simulink model "Mod1_2d_VyP"  (R2019a)
settings: Solver=VariableStepAuto  StartTime=0.0  StopTime=370  MaxStep=0.01  RelTol=1e-3
values from neighbouring files (symbols this model uses):
  a_s = 0.32    [Mod1_2d_VyP_pars.m]
settings Model: Creator=Luis F Guevara G  LastModifiedBy=Luis F Guevara G

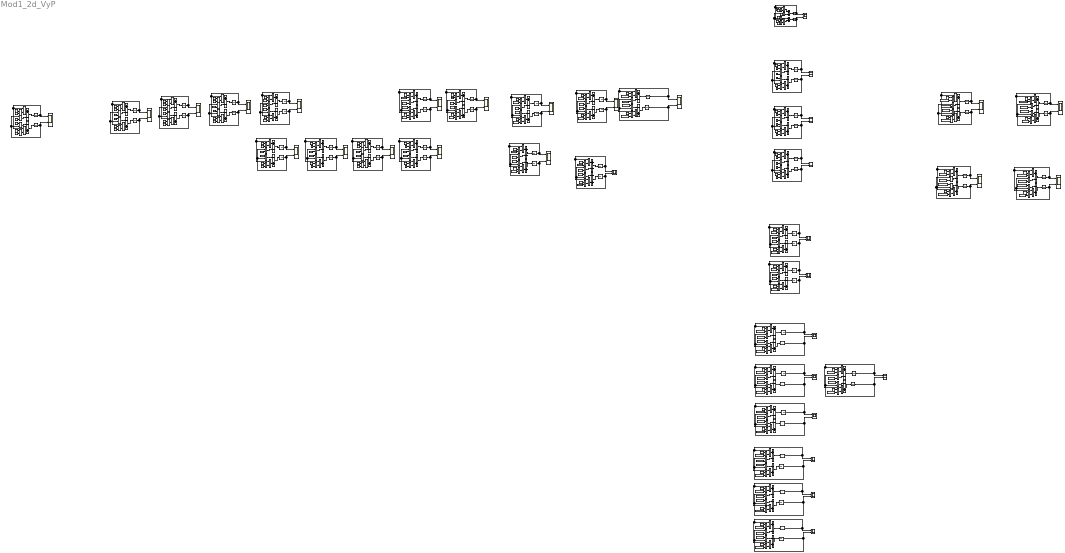
== system Mod1_2d_VyP ==
  note: ESTOS SON DE LOS USADOS
      | PARA EL DOCUMENTO DE LA TESIS
  note: CONSIDEREMOS DATOS DE FERNANDA PARTO #3
      | Peso inicial 515 (Integrador arriba)
      | Desperdicio inicial 44.75 (Integrador abajo)
  note: Cómo controlo la llegada al maximo para
      | luego cambiar el control al llegar al minimo
      | Toca usar automata? omg
  note: OJO SUPER OJO AQUI
  note: Con estos valores, logramos un crecimiento hasta punto maximo
      | y luego decrecimiento hasta que se hace 0
  note: K1=1
      | K2=1
      | K3=1
      | K4= 1
      | a_s = 0.32
  note: P
  note: W
  note: K1=1
      | K2=0.5
      | K3=1
      | K4=0.5
      | a_s = 0.32
  note: P
  note: W
  note: K1=1
      | K2=0.5
      | K3=1
      | K4=0.5
      | a_s = 0.32
  note: P
  note: W
  note: K1=0.5
      | K2=0.25
      | K3=0.5
      | K4=0.25
      | a_s = 0.32
  note: P
  note: W
  note: P
  note: W
  note: K1=1
      | K2=0.3
      | K3=1
      | K4=0.3
      | a_s = 0.32
  note: P
  note: W
  note: K1=1
      | K2=0.51
      | K3=1
      | K4=0.5
      | a_s = 0.32
  note: P
  note: W
  note: Si k4 es mayor a k2 (doble, se indetermina a infinito)
  note: K1=1
      | K2=0.51
      | K3=1
      | K4=0.511
      | a_s = 0.32
  note: OJO SUPER OJO AQUI
  note: Con estos valores, logramos un crecimiento hasta punto maximo
      | y luego decrecimiento hasta que se hace 0
  note: P
  note: W
  note: K1=1
      | K2=0.51
      | K3=1
      | K4=0.509
      | a_s = 0.32
  note: Cómo controlo la llegada al maximo para
      | luego cambiar el control al llegar al minimo
      | Toca usar automata? omg
  note: Con estos valores, logramos un crecimiento hasta punto maximo
      | y luego decrecimiento hasta que se hace 0
  note: W
  note: Cómo controlo la llegada al maximo para
      | luego cambiar el control al llegar al minimo
      | Toca usar automata? omg
  note: OJO SUPER OJO AQUI
  note: P
  note: K1=1
      | K2=0.3
      | K3=1
      | K4=0.29
      | a_s = 0.32
  note: Cómo controlo la llegada al maximo para
      | luego cambiar el control al llegar al minimo
      | Toca usar automata? omg
  note: OJO SUPER OJO AQUI
  note: P
  note: Con estos valores, logramos un crecimiento hasta punto maximo
      | y luego decrecimiento hasta que se hace 0
  note: W
  note: K1=1
      | K2=0.4
      | K3=1
      | K4=0.39
      | a_s = 0.32
  note: W
  note: K1=1
      | K2=0.45
      | K3=1
      | K4=0.44
      | a_s = 0.32
  note: Con estos valores, logramos un crecimiento hasta punto maximo
      | y luego decrecimiento hasta que se hace 0
  note: P
  note: OJO SUPER OJO AQUI
  note: Cómo controlo la llegada al maximo para
      | luego cambiar el control al llegar al minimo
      | Toca usar automata? omg
  note: W
  note: K1=1
      | K2=0.45
      | K3=1
      | K4=0.44
      | a_s = 0.32
  note: Con estos valores, logramos un crecimiento hasta punto maximo
      | y luego decrecimiento hasta que se hace 0 POR ALLA EN T=2K
  note: P
  note: OJO SUPER OJO AQUI
  note: Cómo controlo la llegada al maximo para
      | luego cambiar el control al llegar al minimo
      | Toca usar automata? omg
  note: W
  note: K1=0.3
      | K2=0.7
      | K3=0.2975
      | K4=0.5
      | a_s = 0.32
  note: Con estos valores, logramos un crecimiento hasta punto maximo
      | y luego decrecimiento hasta que se hace 0 POR ALLA EN T=2K
  note: P
  note: OJO SUPER OJO AQUI
  note: Cómo controlo la llegada al maximo para
      | luego cambiar el control al llegar al minimo
      | Toca usar automata? omg
  note: W
  note: K1=0.3
      | K2=0.7
      | K3=0.2975
      | K4=0.5
      | a_s = 0.32
  note: Con estos valores, logramos un crecimiento hasta punto maximo
      | y luego decrecimiento hasta que se hace 0 POR ALLA EN T=2K
  note: P
  note: OJO SUPER OJO AQUI
  note: Cómo controlo la llegada al maximo para
      | luego cambiar el control al llegar al minimo
      | Toca usar automata? omg
  note: CONSIDEREMOS DATOS DE FERNANDA PARTO #3
      | Peso inicial 515 (Integrador arriba)
      | Desperdicio inicial 44.75 (Integrador abajo)
  note: Con estos valores, logramos un crecimiento hasta punto maximo
      | y luego decrecimiento hasta que se hace 0 POR ALLA EN T=2K
  note: Cómo controlo la llegada al maximo para
      | luego cambiar el control al llegar al minimo
      | Toca usar automata? omg
  note: P
  note: W
  note: OJO SUPER OJO AQUI
  note: K1=0.3
      | K2=0.7
      | K3=0.2975
      | K4=0.5
      | a_s = 0.32
  note: W
  note: K1=0.3
      | K2=0.7
      | K3=0.2975
      | K4=0.5
      | a_s = 0.32
  note: Con estos valores, logramos un crecimiento hasta punto maximo
      | y luego decrecimiento hasta que se hace 0 POR ALLA EN T=2K
  note: P
  note: OJO SUPER OJO AQUI
  note: Cómo controlo la llegada al maximo para
      | luego cambiar el control al llegar al minimo
      | Toca usar automata? omg
  note: W
  note: K1=0.3
      | K2=0.7
      | K3=0.2975
      | K4=0.5
      | a_s = 0.32
  note: Con estos valores, logramos un crecimiento hasta punto maximo
      | y luego decrecimiento hasta que se hace 0 POR ALLA EN T=2K
  note: P
  note: OJO SUPER OJO AQUI
  note: Cómo controlo la llegada al maximo para
      | luego cambiar el control al llegar al minimo
      | Toca usar automata? omg
  note: W
  note: P
  note: Parto#3 - Python
      | Fernanda
  note: W
  note: K1=0.2798
      | K2=1
      | K3=0.03218
      | K4=0.1148
      | a_s = 0.32
  note: Con estos valores, logramos un crecimiento hasta punto maximo
      | y luego decrecimiento hasta que se hace 0 POR ALLA EN T=2K
  note: P
  note: OJO SUPER OJO AQUI
  note: Cómo controlo la llegada al maximo para
      | luego cambiar el control al llegar al minimo
      | Toca usar automata? omg
  note: Parto#3 - Python
      | Guapa
  note: W
  note: K1=0.2798
      | K2=1
      | K3=0.03218
      | K4=0.1148
      | a_s = 0.32
  note: Con estos valores, logramos un crecimiento hasta punto maximo
      | y luego decrecimiento hasta que se hace 0 POR ALLA EN T=2K
  note: P
  note: OJO SUPER OJO AQUI
  note: Cómo controlo la llegada al maximo para
      | luego cambiar el control al llegar al minimo
      | Toca usar automata? omg
  note: Parto#3 - Python
      | Juana
  note: W
  note: K1=0.2798
      | K2=1
      | K3=0.03218
      | K4=0.1148
      | a_s = 0.32
  note: Con estos valores, logramos un crecimiento hasta punto maximo
      | y luego decrecimiento hasta que se hace 0 POR ALLA EN T=2K
  note: P
  note: OJO SUPER OJO AQUI
  note: Cómo controlo la llegada al maximo para
      | luego cambiar el control al llegar al minimo
      | Toca usar automata? omg
  note: Parto#3 - Python
      | Leticia
  note: W
  note: K1=0.2798
      | K2=1
      | K3=0.03218
      | K4=0.1148
      | a_s = 0.32
  note: Con estos valores, logramos un crecimiento hasta punto maximo
      | y luego decrecimiento hasta que se hace 0 POR ALLA EN T=2K
  note: P
  note: OJO SUPER OJO AQUI
  note: Cómo controlo la llegada al maximo para
      | luego cambiar el control al llegar al minimo
      | Toca usar automata? omg
  note: P
  note: W
  note: K1=1
      | K2=0.5
      | K3=1
      | K4=0.5
      | a_s = 0.32
  note: P
  note: W
  note: CONSIDEREMOS DATOS DE FERNANDA PARTO #3
      | Peso inicial 515 (Integrador arriba)
      | Desperdicio inicial 44.75 (Integrador abajo)
  note: W
  note: K1=0.3
      | K2=0.7
      | K3=0.2975
      | K4=0.5
      | a_s = 0.32
  note: Con estos valores, logramos un crecimiento hasta punto maximo
      | y luego decrecimiento hasta que se hace 0 POR ALLA EN T=2K
  note: P
  note: OJO SUPER OJO AQUI
  note: Cómo controlo la llegada al maximo para
      | luego cambiar el control al llegar al minimo
      | Toca usar automata? omg
  note: P
  note: W
  note: P
  note: W
  note: P
  note: W
  note: P
  note: W
  note: P
  note: W
  note: P
  note: W
  note: W
  note: P
  note: ESTOS SON DE LOS USADOS
      | PARA EL DOCUMENTO DE LA TESIS
  note: ESTOS SON DE LOS USADOS
      | PARA EL DOCUMENTO DE LA TESIS
  note: Corroboración del ajuste
      | de modelos Python
  note: P
  note: W
  Add{,2,4,6,8,10,12,14,16,18,20,22,24,26,28,30,32,34,36,38,40,42,44,46,48,50,52,54,56,58,60,62,64} (33 alike) : Sum  Inputs=+-
  Add{1,3,5,7,9,11,13,15,17,19,21,23,25,27,29,31,33,35,37,39,41,43,45,47,49,51,53,55,57,59,61,63,65} (33 alike) : Sum  Inputs=-+
  Constant{,1..65} (66 alike) : Constant  Value=a_s
  Integrator{,2,4,6,8,10,12,14,16,18,20,22,24,30,32,34,44,46,48,50,52,54,56,58,60,62,64} (27 alike) : Integrator  InitialCondition=400
  Integrator{1,3,5,7,9,11,13,15,17,19,21,23,25,31,33,35,45,47,49,51,53,55,57,59,61,63,65} (27 alike) : Integrator  InitialCondition=40
  Integrator26 : Integrator  InitialCondition=515
  Integrator27 : Integrator  InitialCondition=44.75
  Integrator28 : Integrator  InitialCondition=515
  Integrator29 : Integrator  InitialCondition=44.75
  Integrator36 : Integrator  InitialCondition=515
  Integrator37 : Integrator  InitialCondition=44.75
  Integrator38 : Integrator  InitialCondition=500
  Integrator39 : Integrator  InitialCondition=44
  Integrator40 : Integrator  InitialCondition=600
  Integrator41 : Integrator  InitialCondition=43.4
  Integrator42 : Integrator  InitialCondition=396
  Integrator43 : Integrator  InitialCondition=36.2
  K1 {1..2,5..12,23} (11 alike) : Constant
  K1 13 : Constant  Value=0.3
  K1 14 : Constant  Value=0.7
  K1 15 : Constant  Value=0.65
  K1 16 : Constant  Value=0.345
  K1 17 : Constant  Value=0.4475
  K1 18 : Constant  Value=0.1563
  K1 19 : Constant  Value=0.27982548
  K1 20 : Constant  Value=0.26049969
  K1 21 : Constant  Value=0.22004866
  K1 22 : Constant  Value=0.30990678
  K1 24 : Constant  Value=0.5
  K1 25 : Constant  Value=0.6
  K1 26 : Constant  Value=0.69
  K1 27 : Constant  Value=0.65
  K1 28 : Constant  Value=0.8
  K1 29 : Constant  Value=0.2
  K1 3 : Constant  Value=0.5
  K1 30 : Constant  Value=0.69
  K1 31 : Constant  Value=0.051755
  K1 32 : Constant  Value=0.95
  K1 4 : Constant  Value=0.5
  P#3 Fer : Scope  NumInputPorts=2
  P#3 Gpa : Scope  NumInputPorts=2
  P#3 Juan : Scope  NumInputPorts=2
  P#3 Leti : Scope  NumInputPorts=2
  Product{,1..197} (198 alike) : Product
  Scope{,3..16,18,20} (17 alike) : Scope  NumInputPorts=2
  igualki : Scope  NumInputPorts=2
  k1 : Constant
  k1MAPk3_k2MAPk4 : Scope  NumInputPorts=2
  k1MAPk3_k2MAPk4_k1Mk2 : Scope  NumInputPorts=2
  k1Mk2_k3Mk4 : Scope  NumInputPorts=2
  k1Mk3_k2Mk4 : Scope  NumInputPorts=2
  k1menk2_k3menk3 : Scope  NumInputPorts=2
  k1menk2_k3menk4 : Scope  NumInputPorts=2
  k1menk3_k2menk1 : Scope  NumInputPorts=2
  k1menk3_k2menk2 : Scope  NumInputPorts=2
  k1menk3_k2menk4 : Scope  NumInputPorts=2
  k2 {,1,3,19,22..23} (6 alike) : Constant
  k2 10 : Constant  Value=0.4
  k2 11 : Constant  Value=0.45
  k2 12 : Constant  Value=0.45
  k2 13 : Constant  Value=0.7
  k2 14 : Constant  Value=0.7
  k2 15 : Constant  Value=0.8
  k2 16 : Constant  Value=0.7
  k2 17 : Constant  Value=0.9
  k2 18 : Constant  Value=0.61
  k2 2 : Constant  Value=0.5
  k2 20 : Constant  Value=0.99999983
  k2 21 : Constant  Value=0.99999824
  k2 24 : Constant  Value=0.5
  k2 25 : Constant  Value=0.69
  k2 26 : Constant  Value=0.6
  k2 27 : Constant  Value=0.8
  k2 28 : Constant  Value=0.9
  k2 29 : Constant  Value=0.69
  k2 30 : Constant  Value=0.69
  k2 31 : Constant  Value=0.051
  k2 32 : Constant  Value=0.8
  k2 4 : Constant  Value=0.25
  k2 5 : Constant  Value=0.3
  k2 6 : Constant  Value=0.51
  k2 7 : Constant  Value=0.51
  k2 8 : Constant  Value=0.51
  k2 9 : Constant  Value=0.3
  k2Mk1_k3MAPk4 : Scope  NumInputPorts=2
  k3 : Constant
  k3 {1..2,5..11,23} (10 alike) : Constant
  k3 12 : Constant  Value=0.9795
  k3 13 : Constant  Value=0.2975
  k3 14 : Constant  Value=0.5
  k3 {15,27..29} (4 alike) : Constant  Value=0.6
  k3 16 : Constant  Value=0.2755
  k3 17 : Constant  Value=0.3755
  k3 18 : Constant  Value=0.051755
  k3 19 : Constant  Value=0.03218680
  k3 20 : Constant  Value=0.02688459
  k3 21 : Constant  Value=0.0169588
  k3 22 : Constant  Value=0.04221679
  k3 24 : Constant  Value=0.7
  k3 25 : Constant  Value=0.65
  k3 26 : Constant  Value=0.8
  k3 3 : Constant  Value=0.5
  k3 30 : Constant  Value=0.7
  k3 31 : Constant  Value=0.61
  k3 32 : Constant  Value=0.9
  k3 4 : Constant  Value=0.5
  k3Mk4_k1MAPk2 : Scope  NumInputPorts=2
  k4 : Constant
  k4 1 : Constant
  k4 10 : Constant  Value=0.39
  k4 11 : Constant  Value=0.44
  k4 12 : Constant  Value=0.44
  k4 {2,6,13..14,16} (5 alike) : Constant  Value=0.5
  k4 {15,27..28,32} (4 alike) : Constant  Value=0.69
  k4 17 : Constant  Value=0.7
  k4 18 : Constant  Value=0.051
  k4 19 : Constant  Value=0.11480125
  k4 20 : Constant  Value=0.10349996
  k4 21 : Constant  Value=0.07715987
  k4 22 : Constant  Value=0.13587340
  k4 23 : Constant
  k4 24 : Constant  Value=0.7
  k4 25 : Constant  Value=0.8
  k4 26 : Constant  Value=0.65
  k4 29 : Constant  Value=0.8
  k4 3 : Constant
  k4 30 : Constant  Value=0.8
  k4 31 : Constant  Value=0.051
  k4 4 : Constant  Value=0.25
  k4 5 : Constant  Value=0.3
  k4 7 : Constant  Value=0.50
  k4 8 : Constant  Value=0.511
  k4 9 : Constant  Value=0.29
  wires:
  Add/1 -> Integrator/1
  Integrator/1 -> Scope/1, Product1/1, Product6/1  "Peso"
  Integrator1/1 -> Product2/1, Product7/2, Scope/2  "Producido"
  Constant/1 -> Product/1
  K1 1/1 -> Product/2
  Product/1 -> Product1/2
  Product1/1 -> Add/1
  k2 1/1 -> Product2/2
  Product2/1 -> Add/2
  k3 1/1 -> Product5/2
  Constant7/1 -> Product5/1
  Product6/1 -> Add1/2
  Product5/1 -> Product6/2
  k4 1/1 -> Product7/1
  Product7/1 -> Add1/1
  Add1/1 -> Integrator1/1
  Add3/1 -> Integrator3/1
  Product11/1 -> Add3/1
  k4 2/1 -> Product11/1
  Product9/1 -> Product10/2
  Product10/1 -> Add3/2
  Constant2/1 -> Product9/1
  k3 2/1 -> Product9/2
  Product8/1 -> Add2/2
  k2 2/1 -> Product8/2
  Product4/1 -> Add2/1
  Product3/1 -> Product4/2
  K1 2/1 -> Product3/2
  Constant1/1 -> Product3/1
  Integrator3/1 -> k1Mk2_k3Mk4/2, Product11/2, Product8/1  "Producido"
  Integrator2/1 -> k1Mk2_k3Mk4/1, Product10/1, Product4/1  "Peso"
  Add2/1 -> Integrator2/1
  Integrator5/1 -> k1menk2_k3menk4/2, Product13/2, Product16/1  "Desp"
  Product15/1 -> Add4/1
  k2 3/1 -> Product16/2
  Add4/1 -> Integrator4/1
  k3 3/1 -> Product17/2
  Product16/1 -> Add4/2
  Constant3/1 -> Product14/1
  K1 3/1 -> Product14/2
  Product17/1 -> Product12/2
  Constant4/1 -> Product17/1
  Product14/1 -> Product15/2
  Integrator4/1 -> Product12/1, Product15/1, k1menk2_k3menk4/1  "Peso"
  Product12/1 -> Add5/2
  k4 3/1 -> Product13/1
  Product13/1 -> Add5/1
  Add5/1 -> Integrator5/1
  Integrator7/1 -> Scope3/2, Product19/2, Product22/1  "Desp"
  Product21/1 -> Add6/1
  k2 4/1 -> Product22/2
  Add6/1 -> Integrator6/1
  k3 4/1 -> Product23/2
  Product22/1 -> Add6/2
  Constant5/1 -> Product20/1
  K1 4/1 -> Product20/2
  Product23/1 -> Product18/2
  Constant6/1 -> Product23/1
  Product20/1 -> Product21/2
  Integrator6/1 -> Product18/1, Product21/1, Scope3/1  "Peso"
  Product18/1 -> Add7/2
  k4 4/1 -> Product19/1
  Product19/1 -> Add7/1
  Add7/1 -> Integrator7/1
  k4 5/1 -> Product25/1
  Product24/1 -> Add9/2
  Product25/1 -> Add9/1
  Add9/1 -> Integrator9/1
  Product26/1 -> Product27/2
  Integrator8/1 -> Product24/1, Product27/1, Scope4/1  "Peso"
  K1 5/1 -> Product26/2
  Constant9/1 -> Product29/1
  k3 5/1 -> Product29/2
  Constant8/1 -> Product26/1
  Add8/1 -> Integrator8/1
  Product28/1 -> Add8/2
  Product29/1 -> Product24/2
  k2 5/1 -> Product28/2
  Product27/1 -> Add8/1
  Integrator9/1 -> Scope4/2, Product25/2, Product28/1  "Desp"
  Integrator11/1 -> Scope5/2, Product31/2, Product34/1  "Desp"
  Constant11/1 -> Product35/1
  Add10/1 -> Integrator10/1
  k2 6/1 -> Product34/2
  k3 6/1 -> Product35/2
  Product35/1 -> Product30/2
  Product33/1 -> Add10/1
  Product34/1 -> Add10/2
  K1 6/1 -> Product32/2
  Constant10/1 -> Product32/1
  Product32/1 -> Product33/2
  Add11/1 -> Integrator11/1
  Integrator10/1 -> Product30/1, Product33/1, Scope5/1  "Peso"
  Product31/1 -> Add11/1
  k4 6/1 -> Product31/1
  Product30/1 -> Add11/2
  Product42/1 -> Add15/2
  Add14/1 -> Integrator14/1
  k2 8/1 -> Product46/2
  Product43/1 -> Add15/1
  k3 8/1 -> Product47/2
  Product45/1 -> Add14/1
  Product46/1 -> Add14/2
  K1 8/1 -> Product44/2
  Product44/1 -> Product45/2
  Constant14/1 -> Product44/1
  Add15/1 -> Integrator15/1
  Integrator15/1 -> Scope7/2, Product43/2, Product46/1  "Desp"
  Product47/1 -> Product42/2
  k4 8/1 -> Product43/1
  Integrator14/1 -> Product42/1, Product45/1, Scope7/1  "Peso"
  Constant15/1 -> Product47/1
  Add13/1 -> Integrator13/1
  Constant12/1 -> Product38/1
  Product38/1 -> Product39/2
  K1 7/1 -> Product38/2
  Product40/1 -> Add12/2
  Product39/1 -> Add12/1
  k3 7/1 -> Product41/2
  k2 7/1 -> Product40/2
  Add12/1 -> Integrator12/1
  Product41/1 -> Product36/2
  Integrator13/1 -> Scope6/2, Product37/2, Product40/1  "Desp"
  Constant13/1 -> Product41/1
  Integrator12/1 -> Product39/1, Product36/1, Scope6/1  "Peso"
  k4 7/1 -> Product37/1
  Product36/1 -> Add13/2
  Product37/1 -> Add13/1
  Integrator16/1 -> Product51/1, Product48/1, Scope8/1  "Peso"
  Constant17/1 -> Product53/1
  Product48/1 -> Add17/2
  k4 9/1 -> Product49/1
  Integrator17/1 -> Scope8/2, Product49/2, Product52/1  "Desp"
  Product53/1 -> Product48/2
  Add16/1 -> Integrator16/1
  Product49/1 -> Add17/1
  k2 9/1 -> Product52/2
  Product52/1 -> Add16/2
  k3 9/1 -> Product53/2
  K1 9/1 -> Product50/2
  Add17/1 -> Integrator17/1
  Product51/1 -> Add16/1
  Constant16/1 -> Product50/1
  Product50/1 -> Product51/2
  Add19/1 -> Integrator19/1
  Constant18/1 -> Product56/1
  Product57/1 -> Add18/1
  K1 10/1 -> Product56/2
  k2 10/1 -> Product58/2
  k3 10/1 -> Product59/2
  Product55/1 -> Add19/1
  Product58/1 -> Add18/2
  Integrator19/1 -> Scope9/2, Product55/2, Product58/1  "Desp"
  Add18/1 -> Integrator18/1
  Product59/1 -> Product54/2
  Product54/1 -> Add19/2
  k4 10/1 -> Product55/1
  Constant19/1 -> Product59/1
  Integrator18/1 -> Product57/1, Product54/1, Scope9/1  "Peso"
  Product56/1 -> Product57/2
  Product60/1 -> Add21/2
  Add20/1 -> Integrator20/1
  Integrator21/1 -> Scope10/2, Product61/2, Product64/1  "Desp"
  k2 11/1 -> Product64/2
  Product61/1 -> Add21/1
  Product63/1 -> Add20/1
  Add21/1 -> Integrator21/1
  Constant20/1 -> Product62/1
  Integrator20/1 -> Product63/1, Product60/1, Scope10/1  "Peso"
  Product64/1 -> Add20/2
  K1 11/1 -> Product62/2
  Product65/1 -> Product60/2
  Constant21/1 -> Product65/1
  k3 11/1 -> Product65/2
  k4 11/1 -> Product61/1
  Product62/1 -> Product63/2
  Product68/1 -> Product69/2
  k4 12/1 -> Product67/1
  k3 12/1 -> Product71/2
  Constant23/1 -> Product71/1
  Product71/1 -> Product66/2
  K1 12/1 -> Product68/2
  Product70/1 -> Add22/2
  Integrator22/1 -> Scope11/1, Product66/1, Product69/1  "Peso"
  Constant22/1 -> Product68/1
  Add23/1 -> Integrator23/1
  Product69/1 -> Add22/1
  Product67/1 -> Add23/1
  k2 12/1 -> Product70/2
  Integrator23/1 -> Product70/1, Product67/2, Scope11/2  "Desp"
  Add22/1 -> Integrator22/1
  Product66/1 -> Add23/2
  Product72/1 -> Add25/2
  Add24/1 -> Integrator24/1
  Integrator25/1 -> Scope12/2, Product73/2, Product76/1  "Desp"
  k2 13/1 -> Product76/2
  Product73/1 -> Add25/1
  Product75/1 -> Add24/1
  Add25/1 -> Integrator25/1
  Constant24/1 -> Product74/1
  Integrator24/1 -> Product75/1, Product72/1, Scope12/1  "Peso"
  Product76/1 -> Add24/2
  K1 13/1 -> Product74/2
  Product77/1 -> Product72/2
  Constant25/1 -> Product77/1
  k3 13/1 -> Product77/2
  k4 13/1 -> Product73/1
  Product74/1 -> Product75/2
  Product80/1 -> Product81/2
  k4 14/1 -> Product79/1
  k3 14/1 -> Product83/2
  Constant27/1 -> Product83/1
  Product83/1 -> Product78/2
  K1 14/1 -> Product80/2
  Product82/1 -> Add26/2
  Integrator26/1 -> Scope13/1, Product78/1, Product81/1  "Peso"
  Constant26/1 -> Product80/1
  Add27/1 -> Integrator27/1
  Product81/1 -> Add26/1
  Product79/1 -> Add27/1
  k2 14/1 -> Product82/2
  Integrator27/1 -> Product82/1, Product79/2, Scope13/2  "Desp"
  Add26/1 -> Integrator26/1
  Product78/1 -> Add27/2
  Add29/1 -> Integrator29/1
  Integrator29/1 -> Product88/1, Product85/2, Scope14/2  "Desp"
  Add28/1 -> Integrator28/1
  Product85/1 -> Add29/1
  Product84/1 -> Add29/2
  k2 15/1 -> Product88/2
  Constant29/1 -> Product89/1
  Product87/1 -> Add28/1
  Product89/1 -> Product84/2
  Integrator28/1 -> Scope14/1, Product84/1, Product87/1  "Peso"
  Product88/1 -> Add28/2
  k3 15/1 -> Product89/2
  K1 15/1 -> Product86/2
  k4 15/1 -> Product85/1
  Constant28/1 -> Product86/1
  Product86/1 -> Product87/2
  Product92/1 -> Product93/2
  k4 16/1 -> Product91/1
  k3 16/1 -> Product95/2
  Constant31/1 -> Product95/1
  Product95/1 -> Product90/2
  K1 16/1 -> Product92/2
  Product94/1 -> Add30/2
  Integrator30/1 -> Scope15/1, Product90/1, Product93/1  "Peso"
  Constant30/1 -> Product92/1
  Add31/1 -> Integrator31/1
  Product93/1 -> Add30/1
  Product91/1 -> Add31/1
  k2 16/1 -> Product94/2
  Integrator31/1 -> Product94/1, Product91/2, Scope15/2  "Desp"
  Add30/1 -> Integrator30/1
  Product90/1 -> Add31/2
  Product96/1 -> Add33/2
  Add32/1 -> Integrator32/1
  Integrator33/1 -> Scope16/2, Product97/2, Product100/1  "Desp"
  k2 17/1 -> Product100/2
  Product97/1 -> Add33/1
  Product99/1 -> Add32/1
  Add33/1 -> Integrator33/1
  Constant32/1 -> Product98/1
  Integrator32/1 -> Product99/1, Product96/1, Scope16/1  "Peso"
  Product100/1 -> Add32/2
  K1 17/1 -> Product98/2
  Product101/1 -> Product96/2
  Constant33/1 -> Product101/1
  k3 17/1 -> Product101/2
  k4 17/1 -> Product97/1
  Product98/1 -> Product99/2
  Product106/1 -> Product107/2
  k4 18/1 -> Product105/1
  k3 18/1 -> Product103/2
  Constant35/1 -> Product103/1
  Product103/1 -> Product104/2
  K1 18/1 -> Product106/2
  Product102/1 -> Add34/2
  Integrator34/1 -> k2Mk1_k3MAPk4/1, Product104/1, Product107/1  "Peso"
  Constant34/1 -> Product106/1
  Add35/1 -> Integrator35/1
  Product107/1 -> Add34/1
  Product105/1 -> Add35/1
  k2 18/1 -> Product102/2
  Integrator35/1 -> k2Mk1_k3MAPk4/2, Product102/1, Product105/2  "Desp"
  Add34/1 -> Integrator34/1
  Product104/1 -> Add35/2
  Product110/1 -> Add37/2
  Add36/1 -> Integrator36/1
  Integrator37/1 -> P#3 Fer/2, Product111/2, Product108/1  "Desp"
  k2 19/1 -> Product108/2
  Product111/1 -> Add37/1
  Product113/1 -> Add36/1
  Add37/1 -> Integrator37/1
  Constant36/1 -> Product112/1
  Integrator36/1 -> Product113/1, Product110/1, P#3 Fer/1  "Peso"
  Product108/1 -> Add36/2
  K1 19/1 -> Product112/2
  Product109/1 -> Product110/2
  Constant37/1 -> Product109/1
  k3 19/1 -> Product109/2
  k4 19/1 -> Product111/1
  Product112/1 -> Product113/2
  Product118/1 -> Product119/2
  k4 20/1 -> Product117/1
  k3 20/1 -> Product115/2
  Constant39/1 -> Product115/1
  Product115/1 -> Product116/2
  K1 20/1 -> Product118/2
  Product114/1 -> Add38/2
  Integrator38/1 -> P#3 Gpa/1, Product116/1, Product119/1  "Peso"
  Constant38/1 -> Product118/1
  Add39/1 -> Integrator39/1
  Product119/1 -> Add38/1
  Product117/1 -> Add39/1
  k2 20/1 -> Product114/2
  Integrator39/1 -> Product117/2, Product114/1, P#3 Gpa/2  "Desp"
  Add38/1 -> Integrator38/1
  Product116/1 -> Add39/2
  Product128/1 -> Add43/2
  Add42/1 -> Integrator42/1
  Integrator43/1 -> P#3 Leti/2, Product129/2, Product126/1  "Desp"
  k2 22/1 -> Product126/2
  Product129/1 -> Add43/1
  Product131/1 -> Add42/1
  Add43/1 -> Integrator43/1
  Constant42/1 -> Product130/1
  Integrator42/1 -> Product131/1, Product128/1, P#3 Leti/1  "Peso"
  Product126/1 -> Add42/2
  K1 22/1 -> Product130/2
  Product127/1 -> Product128/2
  Constant43/1 -> Product127/1
  k3 22/1 -> Product127/2
  k4 22/1 -> Product129/1
  Product130/1 -> Product131/2
  Product124/1 -> Product125/2
  k4 21/1 -> Product123/1
  k3 21/1 -> Product121/2
  Constant41/1 -> Product121/1
  Product121/1 -> Product122/2
  K1 21/1 -> Product124/2
  Product120/1 -> Add40/2
  Integrator40/1 -> P#3 Juan/1, Product125/1, Product122/1  "Peso"
  Constant40/1 -> Product124/1
  Add41/1 -> Integrator41/1
  Product125/1 -> Add40/1
  Product123/1 -> Add41/1
  k2 21/1 -> Product120/2
  Integrator41/1 -> Product123/2, Product120/1, P#3 Juan/2  "Desp"
  Add40/1 -> Integrator40/1
  Product122/1 -> Add41/2
  Add45/1 -> Integrator45/1
  k4/1 -> Product137/1
  "k2 "/1 -> Product134/2
  Integrator45/1 -> Product134/1, Product137/2, Scope18/2  "Producido"
  Integrator44/1 -> Product136/1, Product133/1, Scope18/1  "Peso"
  Constant44/1 -> Product132/1
  k1/1 -> Product132/2
  Add44/1 -> Integrator44/1
  Product133/1 -> Add44/1
  Product134/1 -> Add44/2
  Product132/1 -> Product133/2
  k3/1 -> Product135/2
  Constant45/1 -> Product135/1
  Product135/1 -> Product136/2
  Product137/1 -> Add45/1
  Product136/1 -> Add45/2
  Add46/1 -> Integrator46/1
  Integrator46/1 -> Product141/1, Product138/1, igualki/1  "Peso"
  Integrator47/1 -> Product142/1, Product139/2, igualki/2  "Producido"
  Constant46/1 -> Product140/1
  K1 23/1 -> Product140/2
  Product140/1 -> Product141/2
  Product141/1 -> Add46/1
  k2 23/1 -> Product142/2
  Product142/1 -> Add46/2
  k3 23/1 -> Product143/2
  Constant47/1 -> Product143/1
  Product138/1 -> Add47/2
  Product143/1 -> Product138/2
  k4 23/1 -> Product139/1
  Product139/1 -> Add47/1
  Add47/1 -> Integrator47/1
  Product152/1 -> Product153/2
  Constant50/1 -> Product152/1
  k4 25/1 -> Product151/1
  K1 25/1 -> Product152/2
  k3 25/1 -> Product155/2
  Product154/1 -> Add50/2
  Integrator50/1 -> k1menk3_k2menk4/1, Product153/1, Product150/1  "Peso"
  Product155/1 -> Product150/2
  Product153/1 -> Add50/1
  Constant51/1 -> Product155/1
  k2 25/1 -> Product154/2
  Product150/1 -> Add51/2
  Product151/1 -> Add51/1
  Add50/1 -> Integrator50/1
  Integrator51/1 -> k1menk3_k2menk4/2, Product151/2, Product154/1  "Desp"
  Add51/1 -> Integrator51/1
  Product144/1 -> Add49/2
  Add48/1 -> Integrator48/1
  Integrator49/1 -> Scope20/2, Product145/2, Product148/1  "Desp"
  k2 24/1 -> Product148/2
  Product145/1 -> Add49/1
  Product147/1 -> Add48/1
  Add49/1 -> Integrator49/1
  Constant48/1 -> Product146/1
  Integrator48/1 -> Scope20/1, Product147/1, Product144/1  "Peso"
  Product148/1 -> Add48/2
  K1 24/1 -> Product146/2
  Product149/1 -> Product144/2
  Constant49/1 -> Product149/1
  k3 24/1 -> Product149/2
  k4 24/1 -> Product145/1
  Product146/1 -> Product147/2
  Add53/1 -> Integrator53/1
  Integrator53/1 -> k1menk2_k3menk3/2, Product160/1, Product157/2  "Desp"
  Add52/1 -> Integrator52/1
  Product157/1 -> Add53/1
  Product156/1 -> Add53/2
  k2 26/1 -> Product160/2
  Constant53/1 -> Product161/1
  Product159/1 -> Add52/1
  Product161/1 -> Product156/2
  Integrator52/1 -> k1menk2_k3menk3/1, Product156/1, Product159/1  "Peso"
  Product160/1 -> Add52/2
  k3 26/1 -> Product161/2
  K1 26/1 -> Product158/2
  k4 26/1 -> Product157/1
  Constant52/1 -> Product158/1
  Product158/1 -> Product159/2
  Product164/1 -> Product165/2
  Constant54/1 -> Product164/1
  k4 27/1 -> Product163/1
  K1 27/1 -> Product164/2
  k3 27/1 -> Product167/2
  Product166/1 -> Add54/2
  Integrator54/1 -> k1MAPk3_k2MAPk4/1, Product165/1, Product162/1  "Peso"
  Product167/1 -> Product162/2
  Product165/1 -> Add54/1
  Constant55/1 -> Product167/1
  k2 27/1 -> Product166/2
  Product162/1 -> Add55/2
  Product163/1 -> Add55/1
  Add54/1 -> Integrator54/1
  Integrator55/1 -> k1MAPk3_k2MAPk4/2, Product163/2, Product166/1  "Desp"
  Add55/1 -> Integrator55/1
  Add57/1 -> Integrator57/1
  Integrator57/1 -> k1Mk3_k2Mk4/2, Product172/1, Product169/2  "Desp"
  Add56/1 -> Integrator56/1
  Product169/1 -> Add57/1
  Product168/1 -> Add57/2
  k2 28/1 -> Product172/2
  Constant57/1 -> Product173/1
  Product171/1 -> Add56/1
  Product173/1 -> Product168/2
  Integrator56/1 -> k1Mk3_k2Mk4/1, Product168/1, Product171/1  "Peso"
  Product172/1 -> Add56/2
  k3 28/1 -> Product173/2
  K1 28/1 -> Product170/2
  k4 28/1 -> Product169/1
  Constant56/1 -> Product170/1
  Product170/1 -> Product171/2
  Add59/1 -> Integrator59/1
  Integrator59/1 -> Product178/1, Product175/2, k1menk3_k2menk1/2  "Desp"
  Add58/1 -> Integrator58/1
  Product175/1 -> Add59/1
  Product174/1 -> Add59/2
  k2 29/1 -> Product178/2
  Constant59/1 -> Product179/1
  Product177/1 -> Add58/1
  Product179/1 -> Product174/2
  Integrator58/1 -> Product174/1, Product177/1, k1menk3_k2menk1/1  "Peso"
  Product178/1 -> Add58/2
  k3 29/1 -> Product179/2
  K1 29/1 -> Product176/2
  k4 29/1 -> Product175/1
  Constant58/1 -> Product176/1
  Product176/1 -> Product177/2
  Product182/1 -> Product183/2
  Constant60/1 -> Product182/1
  k4 30/1 -> Product181/1
  K1 30/1 -> Product182/2
  k3 30/1 -> Product185/2
  Product184/1 -> Add60/2
  Integrator60/1 -> k1menk3_k2menk2/1, Product183/1, Product180/1  "Peso"
  Product185/1 -> Product180/2
  Product183/1 -> Add60/1
  Constant61/1 -> Product185/1
  k2 30/1 -> Product184/2
  Product180/1 -> Add61/2
  Product181/1 -> Add61/1
  Add60/1 -> Integrator60/1
  Integrator61/1 -> k1menk3_k2menk2/2, Product181/2, Product184/1  "Desp"
  Add61/1 -> Integrator61/1
  Product188/1 -> Add63/2
  Add62/1 -> Integrator62/1
  Integrator63/1 -> Product189/2, Product186/1, k3Mk4_k1MAPk2/2  "Desp"
  k2 31/1 -> Product186/2
  Product189/1 -> Add63/1
  Product191/1 -> Add62/1
  Add63/1 -> Integrator63/1
  Constant62/1 -> Product190/1
  Integrator62/1 -> Product191/1, Product188/1, k3Mk4_k1MAPk2/1  "Peso"
  Product186/1 -> Add62/2
  K1 31/1 -> Product190/2
  Product187/1 -> Product188/2
  Constant63/1 -> Product187/1
  k3 31/1 -> Product187/2
  k4 31/1 -> Product189/1
  Product190/1 -> Product191/2
  Add65/1 -> Integrator65/1
  Integrator65/1 -> Product196/1, Product193/2, k1MAPk3_k2MAPk4_k1Mk2/2  "Desp"
  Add64/1 -> Integrator64/1
  Product193/1 -> Add65/1
  Product192/1 -> Add65/2
  k2 32/1 -> Product196/2
  Constant65/1 -> Product197/1
  Product195/1 -> Add64/1
  Product197/1 -> Product192/2
  Integrator64/1 -> Product192/1, Product195/1, k1MAPk3_k2MAPk4_k1Mk2/1  "Peso"
  Product196/1 -> Add64/2
  k3 32/1 -> Product197/2
  K1 32/1 -> Product194/2
  k4 32/1 -> Product193/1
  Constant64/1 -> Product194/1
  Product194/1 -> Product195/2
